simulink model "bObserver"  (R2020a)
settings: Solver=VariableStepAuto  StartTime=0.0  StopTime=1.5  FixedStep=0.0005  EnableMultiTasking=on
InitFcn:
  | kp=0.01;
  | ki=0.01;
  | 
  | k=2;
  | em=100000000;
  | GE=1/em;
  | GU=k*ki/GE;
  | GCE=k*kp/GU;
model workspace (MAT data in the model file):
  time = 0.8
values from neighbouring files (symbols this model uses):
  A1 = obj.boostConverter.A1    [BoostController.m]    (also in BoostConverter.m = [-obj.R/obj.L 0;0 -1/(obj.Ro*obj.C)]; BuckBoostConverter.m = [-obj.R/obj.L 0;0 -1/(obj.Ro*obj.C)]; obsmc.m = Asigma{1,1}; workspace_atual.mat = [-16.4  0; 0  -3.50877192982])
  A2 = obj.boostConverter.A2    [BoostController.m]    (also in BoostConverter.m = [-obj.R/obj.L -1/obj.L;1/obj.C -1/(obj.Ro*obj.C)]; BuckBoostConverter.m = [-obj.R/obj.L 1/obj.L;-1/obj.C -1/(obj.Ro*obj.C)]; obsmc.m = Asigma{1,2}; workspace_atual.mat = [-16.4  -200; 350.877192982  -3.50877192982])
  AlarmDeadTime = 0.50    (= 0.5)    [BoostFaultSimulation.m]    (also in workspace_atual.mat; workspace_certo.mat)
  B1 = obj.boostConverter.B1    [BoostController.m]    (also in BoostConverter.m = [1/obj.L;0]; BuckBoostConverter.m = [1/obj.L;0]; obsmc.m = Bsigma{1,1}; workspace_atual.mat = [200 0])
  B1f = [200 0]    [workspace_atual.mat]    (also in workspace_certo.mat)
  B2 = obj.boostConverter.B2    [BoostController.m]    (also in BoostConverter.m = obj.B1; obsmc.m = Bsigma{1,2}; workspace_atual.mat = [200 0]; workspace_certo.mat = [200 0])
  B2f = [200 0]    [workspace_atual.mat]    (also in workspace_certo.mat)
  boost_Amatrices = cat(3,obj.A1,obj.A2)    [BoostConverter.m]    (also in BuckBoostConverter.m; boostResults2Latex.m = boost.A_matrices(); workspace_atual.mat = [-16.4 0 0 -3.50877192982 -16.4 350.877192982 -200 -3.508771; workspace_certo.mat = [-16.4 0 0 -3.50877192982 -16.4 350.877192982 -200 -3.508771)
  boost_parameters = [obj.Ro,obj.R,obj.L,obj.C,obj.u]'    [BoostConverter.m]    (also in BuckBoostConverter.m; boostResults2Latex.m = boost.parameters(); workspace_atual.mat = [100 0.082 0.005 0.00285 190]; workspace_certo.mat = [100 0.082 0.005 0.00285 190])
  C = 1e-3    (= 0.001)    [boostResults2Latex.m]
  CiL = [0 1]    [workspace_atual.mat]    (also in workspace_certo.mat)
  Cmatrix = [1  0; 0  1]    [workspace_atual.mat]    (also in workspace_certo.mat)
  CVc = [1 0]    [workspace_atual.mat]    (also in workspace_certo.mat)
  D1 = [1  0; 0  1]    [workspace_atual.mat]    (also in workspace_certo.mat)
  F_11 = -16.4    [workspace_atual.mat]    (also in workspace_certo.mat)
  F_12 = -4812476.87956    [workspace_atual.mat]    (also in workspace_certo.mat)
  F_21 = -3.50877192982    [workspace_atual.mat]    (also in workspace_certo.mat)
  F_22 = -2.00703596657    [workspace_atual.mat]    (also in workspace_certo.mat)
  FaultClass = 0    [BoostFaultSimulation.m]    (also in workspace_atual.mat = 1; workspace_certo.mat = 1)
  H_1 = 13715.5123667    [workspace_atual.mat]    (also in workspace_certo.mat)
  iLFaultSwitch = 0    [BoostFaultSimulation.m]    (also in workspace_atual.mat; workspace_certo.mat)
  iLFaultTime = 1.70    (= 1.7)    [BoostFaultSimulation.m]    (also in workspace_atual.mat; workspace_certo.mat)
  iLGainFaultFactor = 15    [BoostFaultSimulation.m]    (also in workspace_atual.mat; workspace_certo.mat)
  iLNoiseFaultSwitch = 0    [BoostFaultSimulation.m]    (also in workspace_atual.mat; workspace_certo.mat)
  iLNoiseTime = 1.70    (= 1.7)    [BoostFaultSimulation.m]    (also in workspace_atual.mat; workspace_certo.mat)
  Jth = 2000    [workspace_atual.mat]    (also in workspace_certo.mat)
  L = 1e-3    (= 0.001)    [boostResults2Latex.m]    (also in obsmc.m = sdpvar(3,1,'full'))
  L_11 = -176809.798019    [workspace_atual.mat]    (also in workspace_certo.mat)
  L_12 = -66005538231.6    [workspace_atual.mat]    (also in workspace_certo.mat)
  L_21 = 0.0967961040176    [workspace_atual.mat]    (also in workspace_certo.mat)
  L_22 = 350.985265141    [workspace_atual.mat]    (also in workspace_certo.mat)
  LoadAddSignalSwitch = 1    [BoostFaultSimulation.m]    (also in workspace_atual.mat; workspace_certo.mat)
  LoadAddSwitch = 0    [BoostFaultSimulation.m]    (also in workspace_atual.mat; workspace_certo.mat)
  LoadAddTime = 0.90    (= 0.9)    [BoostFaultSimulation.m]    (also in workspace_atual.mat; workspace_certo.mat)
  LoadRemoveSignalSwitch = 1    [BoostFaultSimulation.m]    (also in workspace_atual.mat; workspace_certo.mat)
  LoadRemoveSwitch = 0    [BoostFaultSimulation.m]    (also in workspace_atual.mat; workspace_certo.mat)
  LoadRemoveTime = 0.90    (= 0.9)    [BoostFaultSimulation.m]    (also in workspace_atual.mat; workspace_certo.mat)
  LobsiL = [1737913.15707 66180.0912281]    [workspace_atual.mat]    (also in workspace_certo.mat)
  LobsVc = [61200 1]    [workspace_atual.mat]    (also in workspace_certo.mat)
  ObsEp = 70    [workspace_atual.mat]    (also in workspace_certo.mat)
  P = value(P)    [BoostController.m]    (also in boostResults2Latex.m = boost.calculateP(); obsmc.m = blkdiag(1/deltaAtilde(1,2),-1/deltaAtilde(2,1),1); workspace_atual.mat = [0.00235275094895  5.25738510027e-05; 5.25738510027e-05  0.0; workspace_certo.mat = [0.00235275094893  5.25738512446e-05; 5.25738512446e-05  0.0)
  Q_1 = [13715.5123667  1; 1  0]    [workspace_atual.mat]    (also in workspace_certo.mat)
  Q_2 = [1  0; 0.00750867981628  1]    [workspace_atual.mat]    (also in workspace_certo.mat)
  R = 0.1    [boostResults2Latex.m]    (also in workspace_atual.mat = 0.082; workspace_certo.mat = 0.082)
  ReconfigSwitch = 0    [BoostFaultSimulation.m]    (also in workspace_atual.mat; workspace_certo.mat)
  ReconfigTime = 1.707    [BoostFaultSimulation.m]    (also in workspace_atual.mat; workspace_certo.mat)
  rho = 5    [workspace_atual.mat]    (also in workspace_certo.mat)
  RMSfrequency = 47.61    [BoostFaultSimulation.m]    (also in workspace_atual.mat; workspace_certo.mat)
  Ro = 100    [BoostFaultSimulation.m]    (also in boostResults2Latex.m = 10; workspace_atual.mat; workspace_certo.mat)
  Smep = 80    [workspace_atual.mat]    (also in workspace_certo.mat)
  SourceAddSignalSwitch = 1    [BoostFaultSimulation.m]    (also in workspace_atual.mat; workspace_certo.mat)
  SourceAddSwitch = 0    [BoostFaultSimulation.m]    (also in workspace_atual.mat; workspace_certo.mat)
  SourceAddTime = 0.90    (= 0.9)    [BoostFaultSimulation.m]    (also in workspace_atual.mat; workspace_certo.mat)
  SourceAddVoltage = obj.SourceAddFactor*obj.u    [BoostFaultSimulation.m]    (also in workspace_atual.mat = 19; workspace_certo.mat = 19)
  SourceRemoveSignalSwitch = 1    [BoostFaultSimulation.m]    (also in workspace_atual.mat; workspace_certo.mat)
  SourceRemoveSwitch = 0    [BoostFaultSimulation.m]    (also in workspace_atual.mat; workspace_certo.mat)
  SourceRemoveTime = 0.90    (= 0.9)    [BoostFaultSimulation.m]    (also in workspace_atual.mat; workspace_certo.mat)
  SourceRemoveVoltage = obj.SourceRemoveFactor*obj.u    [BoostFaultSimulation.m]    (also in workspace_atual.mat = 19; workspace_certo.mat = 19)
  T_1 = [1 -13715.5123667]    [workspace_atual.mat]    (also in workspace_certo.mat)
  T_2 = [-0.00750867981628 1]    [workspace_atual.mat]    (also in workspace_certo.mat)
  ueq = 0.5    [workspace_atual.mat]    (also in workspace_certo.mat)
  uf = 190    [workspace_atual.mat]    (also in workspace_certo.mat)
  VcFaultSwitch = 0    [BoostFaultSimulation.m]    (also in workspace_atual.mat; workspace_certo.mat)
  VcFaultTime = 1.70    (= 1.7)    [BoostFaultSimulation.m]    (also in workspace_atual.mat; workspace_certo.mat)
  VcGainFaultFactor = 15    [BoostFaultSimulation.m]    (also in workspace_atual.mat; workspace_certo.mat)
  VcNoiseFaultSwitch = 0    [BoostFaultSimulation.m]    (also in workspace_atual.mat; workspace_certo.mat)
  VcNoiseTime = 1.70    (= 1.7)    [BoostFaultSimulation.m]    (also in workspace_atual.mat; workspace_certo.mat)
  ve = 380    [BoostFaultSimulation.m]    (also in boostResults2Latex.m = 100; workspace_atual.mat; workspace_certo.mat)
  x_e = [ie;ve]    [BoostConverter.m]    (also in BuckBoostConverter.m)
  xe = obj.boostConverter.equilibriumstate(ve)    [BoostController.m]    (also in workspace_atual.mat = [7.62509288104 380]; workspace_certo.mat = [7.62509288104 380])
undefined symbols (not defined in the file or in its folder): Atilde1, Atilde2, B1u, Ctilde1, Dtilde1, Dtilde2, F, F1, G, G1, MAXnet, MINnet
libraries: neural x36, powerlib x34, dspstat3 x11, PhdLibrary x10, simulink x7, dspmtrx3 x6, powerlib_meascontrol x4, dspmathops x4
(part 3 of 6)

== system bObserver/ROSLSO/Bank of ROSLSO/z1 ==
  y_f1 : Inport
  sigma : Inport  Port=2
  Constant : Constant  Value=F_11  VectorParams1D=off
  Constant10 : Constant  Value=T_1  VectorParams1D=off
  Constant2 : Constant  Value=F_12  VectorParams1D=off
  Constant4 : Constant  Value=L_11  VectorParams1D=off
  Constant5 : Constant  Value=L_12  VectorParams1D=off
  Integral : Subsystem
  Matrix Multiply{,1..4} (5 alike) : Product  Multiplication=Matrix(*)
  MatrizesA8 : Constant  Value=B1u  VectorParams1D=off
  Sum : Sum  Inputs=|+++
  Sum1 : Sum  Inputs=|+++
  Switch1 : Switch  Criteria=u2 ~= 0
  z : Outport
  wires:
  sigma/1 -> Switch1/2
  Switch1/1 -> Integral/1(z_dot)  "z"
  Sum/1 -> [sys1]
  Sum1/1 -> [sys2]
  Integral/1(z) -> [z], z/1
  y_f1/1 -> Matrix Multiply2/2, Matrix Multiply/2
  MatrizesA8/1 -> Matrix Multiply1/2
  Constant10/1 -> Matrix Multiply1/1
  Matrix Multiply1/1 -> [TBu]
  Matrix Multiply/1 -> [Ly1]
  Matrix Multiply2/1 -> [Ly2]
  Matrix Multiply3/1 -> [Fz1]
  Constant/1 -> Matrix Multiply3/1
  Matrix Multiply4/1 -> [Fz2]
  Constant2/1 -> Matrix Multiply4/1
  [z] -> Matrix Multiply4/2
  [Fz1] -> Sum/1
  [Fz2] -> Sum1/1
  [z] -> Matrix Multiply3/2
  [sys1] -> Switch1/1
  [sys2] -> Switch1/3
  [TBu] -> Sum/2
  [TBu] -> Sum1/2
  [Ly2] -> Sum1/3
  [Ly1] -> Sum/3
  Constant4/1 -> Matrix Multiply/1
  Constant5/1 -> Matrix Multiply2/1

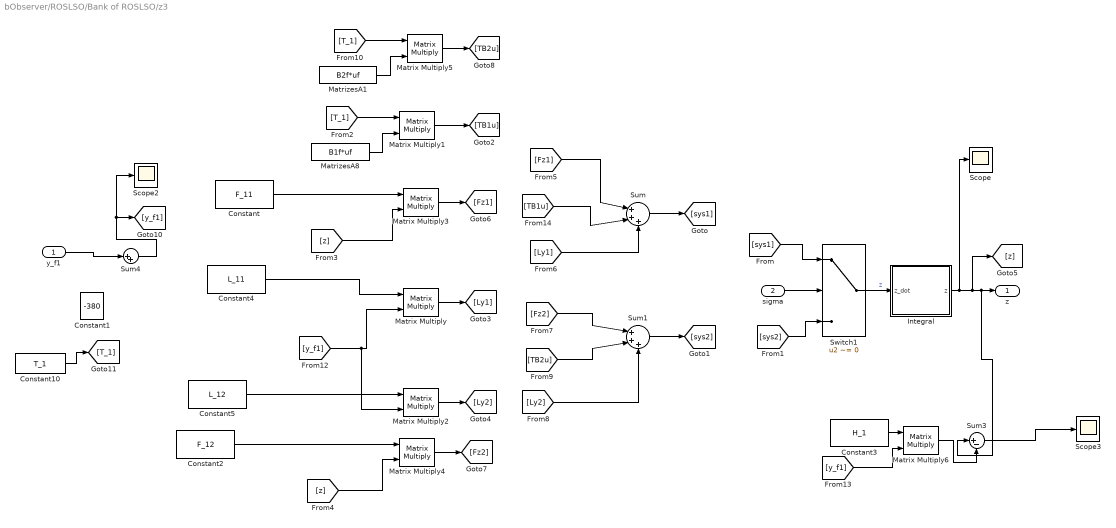
== system bObserver/ROSLSO/Bank of ROSLSO/z3 ==
  y_f1 : Inport
  sigma : Inport  Port=2
  Constant : Constant  Value=F_11  VectorParams1D=off
  Constant1 : Constant  Value=-380
  Constant10 : Constant  Value=T_1  VectorParams1D=off
  Constant2 : Constant  Value=F_12  VectorParams1D=off
  Constant3 : Constant  Value=H_1  VectorParams1D=off
  Constant4 : Constant  Value=L_11  VectorParams1D=off
  Constant5 : Constant  Value=L_12  VectorParams1D=off
  Integral : Subsystem
  Matrix Multiply{,1..6} (7 alike) : Product  Multiplication=Matrix(*)
  MatrizesA1 : Constant  Value=B2f*uf  VectorParams1D=off
  MatrizesA8 : Constant  Value=B1f*uf  VectorParams1D=off
  Scope : Scope
  Scope2 : Scope
  Scope3 : Scope
  Sum : Sum  Inputs=|+++
  Sum1 : Sum  Inputs=|+++
  Sum3 : Sum  Inputs=|+-
  Sum4 : Sum  Inputs=|++
  Switch1 : Switch  Criteria=u2 ~= 0
  z : Outport
  wires:
  sigma/1 -> Switch1/2
  Switch1/1 -> Integral/1(z_dot)  "z"
  Sum/1 -> [sys1]
  Sum1/1 -> [sys2]
  Integral/1(z) -> Scope/1, [z], Sum3/1, z/1
  MatrizesA8/1 -> Matrix Multiply1/2
  [T_1] -> Matrix Multiply1/1
  Matrix Multiply1/1 -> [TB1u]
  Matrix Multiply/1 -> [Ly1]
  Matrix Multiply2/1 -> [Ly2]
  Matrix Multiply3/1 -> [Fz1]
  Matrix Multiply4/1 -> [Fz2]
  [z] -> Matrix Multiply4/2
  [Fz1] -> Sum/1
  [Fz2] -> Sum1/1
  [z] -> Matrix Multiply3/2
  [sys1] -> Switch1/1
  [sys2] -> Switch1/3
  [TB2u] -> Sum1/2
  [Ly2] -> Sum1/3
  [Ly1] -> Sum/3
  Constant4/1 -> Matrix Multiply/1
  Constant3/1 -> Matrix Multiply6/1
  [y_f1] -> Matrix Multiply2/2, Matrix Multiply/2
  [y_f1] -> Matrix Multiply6/2
  Matrix Multiply6/1 -> Sum3/2
  Sum3/1 -> Scope3/1
  Constant/1 -> Matrix Multiply3/1
  Constant2/1 -> Matrix Multiply4/1
  Constant5/1 -> Matrix Multiply2/1
  y_f1/1 -> Sum4/1
  Sum4/1 -> Scope2/1, [y_f1]
  [TB1u] -> Sum/2
  Constant10/1 -> [T_1]
  [T_1] -> Matrix Multiply5/1
  Matrix Multiply5/1 -> [TB2u]
  MatrizesA1/1 -> Matrix Multiply5/2

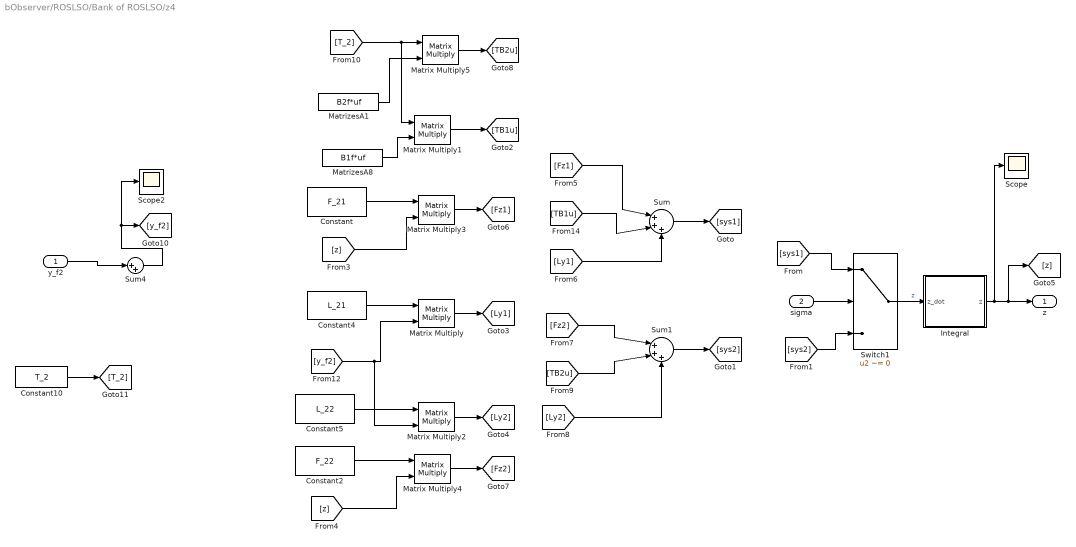
== system bObserver/ROSLSO/Bank of ROSLSO/z4 ==
  y_f2 : Inport
  sigma : Inport  Port=2
  Constant : Constant  Value=F_21  VectorParams1D=off
  Constant10 : Constant  Value=T_2  VectorParams1D=off
  Constant2 : Constant  Value=F_22  VectorParams1D=off
  Constant4 : Constant  Value=L_21  VectorParams1D=off
  Constant5 : Constant  Value=L_22  VectorParams1D=off
  Integral : Subsystem
  Matrix Multiply{,1..5} (6 alike) : Product  Multiplication=Matrix(*)
  MatrizesA1 : Constant  Value=B2f*uf  VectorParams1D=off
  MatrizesA8 : Constant  Value=B1f*uf  VectorParams1D=off
  Scope : Scope
  Scope2 : Scope
  Sum : Sum  Inputs=|+++
  Sum1 : Sum  Inputs=|+++
  Sum4 : Sum  Inputs=|++
  Switch1 : Switch  Criteria=u2 ~= 0
  z : Outport
  wires:
  sigma/1 -> Switch1/2
  Switch1/1 -> Integral/1(z_dot)  "z"
  Sum/1 -> [sys1]
  Sum1/1 -> [sys2]
  Integral/1(z) -> Scope/1, [z], z/1
  MatrizesA8/1 -> Matrix Multiply1/2
  [T_2] -> Matrix Multiply1/1, Matrix Multiply5/1
  Matrix Multiply1/1 -> [TB1u]
  Matrix Multiply/1 -> [Ly1]
  Matrix Multiply2/1 -> [Ly2]
  Matrix Multiply3/1 -> [Fz1]
  Matrix Multiply4/1 -> [Fz2]
  [z] -> Matrix Multiply4/2
  [Fz1] -> Sum/1
  [Fz2] -> Sum1/1
  [z] -> Matrix Multiply3/2
  [sys1] -> Switch1/1
  [sys2] -> Switch1/3
  Constant4/1 -> Matrix Multiply/1
  [y_f2] -> Matrix Multiply2/2, Matrix Multiply/2
  Constant/1 -> Matrix Multiply3/1
  Constant2/1 -> Matrix Multiply4/1
  Constant5/1 -> Matrix Multiply2/1
  y_f2/1 -> Sum4/1
  Sum4/1 -> Scope2/1, [y_f2]
  Constant10/1 -> [T_2]
  Matrix Multiply5/1 -> [TB2u]
  MatrizesA1/1 -> Matrix Multiply5/2
  [TB1u] -> Sum/2
  [TB2u] -> Sum1/2
  [Ly1] -> Sum/3
  [Ly2] -> Sum1/3

== system bObserver/ROSLSO/Bank of ROSMO/Subsystem ==
  y : Inport
  C : Inport  Port=2
  y_hat : Inport  Port=3
  "    1" : Constant  Value=ObsEp
  Product : Product  Multiplication=Matrix(*)
  SlidingSurface : Subsystem
  Subtract : Sum  Inputs=+-
  error : Outport
  wires:
  Subtract/1 -> SlidingSurface/1(S)  "y-y_hat"
  Product/1 -> Subtract/1
  "    1"/1 -> SlidingSurface/2(ep)
  SlidingSurface/1(d) -> error/1
  y_hat/1 -> Subtract/2
  C/1 -> Product/1
  y/1 -> Product/2

== system bObserver/ROSLSO/Bank of ROSMO/Subsystem1 ==
  y : Inport
  C : Inport  Port=2
  y_hat : Inport  Port=3
  "    1" : Constant  Value=ObsEp
  Product : Product  Multiplication=Matrix(*)
  SlidingSurface : Subsystem
  Subtract : Sum  Inputs=+-
  error : Outport
  wires:
  Subtract/1 -> SlidingSurface/1(S)  "y-y_hat"
  Product/1 -> Subtract/1
  "    1"/1 -> SlidingSurface/2(ep)
  SlidingSurface/1(d) -> error/1
  y_hat/1 -> Subtract/2
  C/1 -> Product/1
  y/1 -> Product/2

== system bObserver/ROSLSO/Bank of ROSMO/Vc OBserver ==
  ObserverError : Inport
  C : Inport  Port=2
  sigma : Inport  Port=3
  Constant : Constant  Value=LobsVc
  Product2 : Product  Multiplication=Matrix(*)
  calc_x_hat : Subsystem
  x_hat : Outport
  y_hat : Outport  Port=2
  wires:
  sigma/1 -> calc_x_hat/1(sigma)
  calc_x_hat/1(x_hat) -> Product2/2, x_hat/1
  Product2/1 -> y_hat/1
  C/1 -> Product2/1
  ObserverError/1 -> calc_x_hat/2(rsign)
  Constant/1 -> calc_x_hat/3(Lobs)

== system bObserver/ROSLSO/Bank of ROSMO/iL Observer ==
  C : Inport
  ObserverError : Inport  Port=2
  sigma : Inport  Port=3
  Constant8 : Constant  Value=LobsiL
  Product2 : Product  Multiplication=Matrix(*)
  calc_x_hat : Subsystem
  x_hat : Outport
  y_hat : Outport  Port=2
  wires:
  sigma/1 -> calc_x_hat/1(sigma)
  calc_x_hat/1(x_hat) -> Product2/2, x_hat/1
  Product2/1 -> y_hat/1
  C/1 -> Product2/1
  ObserverError/1 -> calc_x_hat/2(rsign)
  Constant8/1 -> calc_x_hat/3(Lobs)

== system bObserver/ROSLSO/Boost Converter/Integral ==
  x_dot : Inport
  Ground : Ground
  Ground1 : Ground
  IC : InitialCondition  Value=[0;0]
  Integrator1 : Integrator  InitialConditionSource=external  InitialCondition=[-x_e; 0; 0]
  Mux : Mux  Inputs=2
  x : Outport
  wires:
  x_dot/1 -> Integrator1/1
  Integrator1/1 -> x/1
  IC/1 -> Integrator1/2
  Ground1/1 -> Mux/2
  Ground/1 -> Mux/1
  Mux/1 -> IC/1

== system bObserver/ROSLSO/Chaveado_fixo1/Controlador Chavead ==
  Ve : Inport
  x : Inport  Port=2
  MatirxControle : Subsystem
  Matrix P : Constant  Value=P
  Matrizes A : Constant  Value=boost_Amatrices
  Parametros do Boost : Constant  Value=boost_parameters
  sigma : Outport
  x_e : Outport  Port=2
  i_e : Outport  Port=3
  wires:
  Parametros do Boost/1 -> MatirxControle/1("boost_parameters ")
  Matrizes A/1 -> MatirxControle/2(boost_Amatrices)
  Matrix P/1 -> MatirxControle/3(P)
  x/1 -> MatirxControle/5(x)
  Ve/1 -> MatirxControle/4(ve)
  MatirxControle/1(sigma) -> sigma/1
  MatirxControle/2(x_e) -> x_e/1
  MatirxControle/3(i_e) -> i_e/1

== system bObserver/ROSLSO/Controlador1/SlidingSurface ==
  S : Inport
  ep : Inport  Port=2
  Abs : Abs
  GreaterThan : RelationalOperator  Operator=>  OutDataTypeStr=boolean  RndMeth=Simplest
  If : If  IfExpression=u1 ~= 0
  If Action Subsystem : Subsystem  TreatAsAtomicUnit=on
  If Action Subsystem2 : Subsystem  TreatAsAtomicUnit=on
  Merge1 : Merge
  d : Outport
  wires:
  If Action Subsystem2/1(d) -> Merge1/2
  [S] -> If Action Subsystem/1(S), If Action Subsystem2/1(S)
  If/2 -> If Action Subsystem2/Action
  If/1 -> If Action Subsystem/Action
  [ep] -> If Action Subsystem2/2(ep)
  S/1 -> [S], Abs/1
  If Action Subsystem/1(d) -> Merge1/1
  Abs/1 -> GreaterThan/1
  GreaterThan/1 -> If/1
  Merge1/1 -> d/1
  ep/1 -> [ep], GreaterThan/2

== system bObserver/ROSLSO/Fault Diagnostics/AntiFalseAlarm ==
  PRNN : Inport
  Alarm : Inport  Port=2
  Constant7 : Constant
  FaultDetecition1 : Switch  Criteria=u2 > Threshold
  Product1 : Product
  Step1 : Step  Time=AlarmDeadTime  SampleTime=0
  FaultClass : Outport
  AlarmOut : Outport  Port=2
  wires:
  PRNN/1 -> FaultDetecition1/1
  Constant7/1 -> FaultDetecition1/3
  Step1/1 -> Product1/1
  Alarm/1 -> Product1/2
  FaultDetecition1/1 -> FaultClass/1
  Product1/1 -> AlarmOut/1, FaultDetecition1/2

== system bObserver/ROSLSO/Fault Diagnostics/Augmented Error Generator ==
  e : Inport
  Mux : Mux  Inputs=2
  z1 : Subsystem
  e_tilde : Outport
  wires:
  z1/1(z) -> Mux/2
  Mux/1 -> e_tilde/1
  e/1 -> Mux/1, z1/1(z_dot)

== system bObserver/ROSLSO/Fault Diagnostics/ErrorGenerator ==
  y_e_tilde : Inport
  y_e_tilde_hat : Inport  Port=2
  AND : Logic  IconShape=distinctive  AllPortsSameDT=off  OutDataTypeStr=boolean
  Compare To Zero : simulink/Logic and Bit Operations/Compare To Zero  relop=~=  OutDataTypeStr=boolean
  Constant1 : Constant  Value=[0;0]
  Demux : Demux  Outputs=2
  If : If  IfExpression=u1 ~= 0
  If Action Subsystem : Subsystem  TreatAsAtomicUnit=on
  If Action Subsystem1 : Subsystem  TreatAsAtomicUnit=on
  Merge : Merge  InitialOutput=[0;0]
  Sum : Sum  Inputs=|+-
  e_y : Outport
  v : Outport  Port=2
  wires:
  y_e_tilde/1 -> Sum/1
  y_e_tilde_hat/1 -> Sum/2
  Sum/1 -> Compare To Zero/1, e_y/1, [e_y]
  If/1 -> If Action Subsystem/Action
  If/2 -> If Action Subsystem1/Action
  [e_y] -> If Action Subsystem/1(e_y)
  Constant1/1 -> If Action Subsystem1/1(e_y)
  If Action Subsystem/1(v) -> Merge/1
  If Action Subsystem1/1(v) -> Merge/2
  Demux/1 -> AND/1
  Demux/2 -> AND/2
  AND/1 -> If/1
  Merge/1 -> v/1
  Compare To Zero/1 -> Demux/1

== system bObserver/ROSLSO/Fault Diagnostics/Fault Identification Neural Netowrk ==
  netInputs : Inport
  Constant : Constant  Commented=on  Value=MAXnet
  Constant1 : Constant  Commented=on  Value=[0;0;0]
  Constant4 : Constant  Commented=on  Value=MINnet
  Demux : Demux  Commented=on  Outputs=3
  Demux1 : Demux  Commented=on  Outputs=3
  Demux2 : Demux  Commented=on  Outputs=3
  Maximum : dspstat3/Maximum  operation=maximum  fcn=Value and Index  indexBase=One  operateOver=Each column  Dimension=1  InputProcessing=Columns as channels (frame based)  reset=None  roiEnable=off  roiType=Rectangles  roiPortion=Entire ROI  roiOutput=Individual statistics for each ROI  roiFlag=off  roundingMode=Floor  overflowMode=off  accumDataTypeStr=Inherit: Same as product output  accumLastDataTypeStr=Inherit: Same as product output
  Median Filter : dspstat3/Median Filter  Commented=on  WindowLength=1  SimulateUsing=Code generation
      settings: SourceProductBaseCode=DS
  Mux : Mux  Commented=on  Inputs=3
  Pattern Recognition Neural Network1 : Subsystem
      mask help: Pattern Recognition Neural Network
      mask Display: e = 0.06;c1 = [120 150 230]/255;c2 = ([120 150 230]+0)/383;c3 = ([120 150 230]+128)/383;patch([0 1 1 0],[0 0 1 1],c1);patch([0 1 1 1-e 1-e 0+e],[0 0 1 1-e 0+e 0+e],c2);patch([0 0 1 1-e 0+e 0+e],[0 1 1 1-e 1-e 0+e],c3);plot([0 1 1 0 0],[0 0 1 1 0]);fprintf('NNET');port_label('input',1,' Input');port_label('output',1,'Output ');
  Scope : Scope
  Scope1 : Scope
  Subsystem : Subsystem  Commented=on
  Subsystem1 : Subsystem  Commented=on
  Subsystem2 : Subsystem  Commented=on
  Terminator : Terminator
  netOutputs : Outport
  wires:
  Maximum/1 -> Terminator/1
  Maximum/2 -> Scope1/1, netOutputs/1, Scope/1
  Constant/1 -> Demux/1
  Demux2/1 -> Subsystem/1(input)
  Demux1/1 -> Subsystem/2(min)
  Demux/1 -> Subsystem/3(max)
  Demux1/2 -> Subsystem1/2(min)
  Demux/2 -> Subsystem1/3(max)
  Demux2/2 -> Subsystem1/1(input)
  Demux/3 -> Subsystem2/3(max)
  Demux1/3 -> Subsystem2/2(min)
  Demux2/3 -> Subsystem2/1(input)
  Subsystem/1(Out1) -> Mux/1
  Subsystem1/1(Out1) -> Mux/2
  Subsystem2/1(Out1) -> Mux/3
  Constant4/1 -> Demux1/1
  netInputs/1 -> Pattern Recognition Neural Network1/1(Input)
  Pattern Recognition Neural Network1/1(Output) -> Maximum/1

== system bObserver/ROSLSO/Fault Diagnostics/Residual Generator2 ==
  e_y : Inport
  Matrix Square1 : dspmtrx3/Matrix Square  OutMin=[]  OutMax=[]
      settings: SourceProductBaseCode=DS
  Moving RMS : dspstat3/Moving RMS  Method=Sliding window  ForgettingFactorPort=off  SpecifyWindowLength=on  WindowLength=RMSfrequency/10  ForgettingFactor=0.9  SimulateUsing=Code generation
      settings: SourceProductBaseCode=DS
  Sqrt2 : Sqrt  SaturateOnIntegerOverflow=on
  RMS : Outport
  wires:
  Matrix Square1/1 -> Sqrt2/1
  e_y/1 -> Matrix Square1/1
  Sqrt2/1 -> Moving RMS/1
  Moving RMS/1 -> RMS/1

== system bObserver/ROSLSO/Fault Diagnostics/Sliding Mode Observer 5 ==
  ey : Inport
  v : Inport  Port=2
  sigma : Inport  Port=3
  C : Constant  Value=Ctilde1
  ObserverDynamics : Subsystem
  Product : Product  Multiplication=Matrix(*)
  ey_out : Outport
  y_e_tilde_hat : Outport  Port=2
  wires:
  Product/1 -> y_e_tilde_hat/1
  C/1 -> Product/1
  ObserverDynamics/1(e_tilde_hat) -> Product/2
  sigma/1 -> ObserverDynamics/3(sigma)
  ey/1 -> ey_out/1, ObserverDynamics/1(ey)
  v/1 -> ObserverDynamics/2(v)

== system bObserver/ROSLSO/Fault Diagnostics/Subsystem9 ==
  x : Inport
  Demux : Demux  Outputs=2
  Residual Generator2 : Subsystem
  Terminator : Terminator
  VcRMS : Outport
  wires:
  x/1 -> Demux/1
  Demux/2 -> Residual Generator2/1(e_y)
  Residual Generator2/1(RMS) -> VcRMS/1
  Demux/1 -> Terminator/1

== system bObserver/ROSMO_L1/Augmented Error Generator/z1 ==
  z_dot : Inport
  Constant1 : Constant  Value=[0;0]  VectorParams1D=off
  Gain2 : Gain  Gain=Cmatrix  Multiplication=Matrix(K*u) (u vector)
  Integrator6 : Integrator  InitialConditionSource=external
  z : Outport
  wires:
  Gain2/1 -> Integrator6/1
  Integrator6/1 -> z/1
  z_dot/1 -> Gain2/1
  Constant1/1 -> Integrator6/2

== system bObserver/ROSMO_L1/Boost Converter/Integral ==
  x_dot : Inport
  Ground : Ground
  Ground1 : Ground
  IC : InitialCondition  Value=[0;0]
  Integrator1 : Integrator  InitialConditionSource=external  InitialCondition=[-x_e; 0; 0]
  Mux : Mux  Inputs=2
  x : Outport
  wires:
  x_dot/1 -> Integrator1/1
  Integrator1/1 -> x/1
  IC/1 -> Integrator1/2
  Ground1/1 -> Mux/2
  Ground/1 -> Mux/1
  Mux/1 -> IC/1

== system bObserver/ROSMO_L1/Controlador2/SlidingSurface ==
  S : Inport
  ep : Inport  Port=2
  Abs : Abs
  GreaterThan : RelationalOperator  Operator=>  OutDataTypeStr=boolean  RndMeth=Simplest
  If : If  IfExpression=u1 ~= 0
  If Action Subsystem : Subsystem  TreatAsAtomicUnit=on
  If Action Subsystem2 : Subsystem  TreatAsAtomicUnit=on
  Merge1 : Merge
  d : Outport
  wires:
  If Action Subsystem2/1(d) -> Merge1/2
  [S] -> If Action Subsystem/1(S), If Action Subsystem2/1(S)
  If/2 -> If Action Subsystem2/Action
  If/1 -> If Action Subsystem/Action
  [ep] -> If Action Subsystem2/2(ep)
  S/1 -> [S], Abs/1
  If Action Subsystem/1(d) -> Merge1/1
  Abs/1 -> GreaterThan/1
  GreaterThan/1 -> If/1
  Merge1/1 -> d/1
  ep/1 -> [ep], GreaterThan/2

== system bObserver/ROSMO_L1/SMO/ErrorGenerator ==
  y_e_tilde : Inport
  y_e_tilde_hat : Inport  Port=2
  AND : Logic  IconShape=distinctive  AllPortsSameDT=off  OutDataTypeStr=boolean
  Compare To Zero : simulink/Logic and Bit Operations/Compare To Zero  relop=~=  OutDataTypeStr=boolean
  Constant1 : Constant  Value=[0;0]
  Demux : Demux  Outputs=2
  If : If  IfExpression=u1 ~= 0
  If Action Subsystem : Subsystem  TreatAsAtomicUnit=on
  If Action Subsystem1 : Subsystem  TreatAsAtomicUnit=on
  Merge : Merge  InitialOutput=[0;0]
  Sum : Sum  Inputs=|+-
  e_y : Outport
  v : Outport  Port=2
  wires:
  y_e_tilde/1 -> Sum/1
  y_e_tilde_hat/1 -> Sum/2
  Sum/1 -> Compare To Zero/1, e_y/1, [e_y]
  If/1 -> If Action Subsystem/Action
  If/2 -> If Action Subsystem1/Action
  [e_y] -> If Action Subsystem/1(e_y)
  Constant1/1 -> If Action Subsystem1/1(e_y)
  If Action Subsystem/1(v) -> Merge/1
  If Action Subsystem1/1(v) -> Merge/2
  Demux/1 -> AND/1
  Demux/2 -> AND/2
  AND/1 -> If/1
  Merge/1 -> v/1
  Compare To Zero/1 -> Demux/1

== system bObserver/ROSMO_L1/SMO/Sliding Mode Observer 5 ==
  ey : Inport
  v : Inport  Port=2
  sigma : Inport  Port=3
  C : Constant  Value=Ctilde1
  ObserverDynamics : Subsystem
  Product : Product  Multiplication=Matrix(*)
  ey_out : Outport
  y_e_tilde_hat : Outport  Port=2
  wires:
  Product/1 -> y_e_tilde_hat/1
  C/1 -> Product/1
  ObserverDynamics/1(e_tilde_hat) -> Product/2
  sigma/1 -> ObserverDynamics/3(sigma)
  ey/1 -> ey_out/1, ObserverDynamics/1(ey)
  v/1 -> ObserverDynamics/2(v)

== system bObserver/ROSMO_ROSLSO/Augmented Error Generator/z1 ==
  z_dot : Inport
  Constant1 : Constant  Value=[0;0]  VectorParams1D=off
  Gain2 : Gain  Gain=Cmatrix  Multiplication=Matrix(K*u) (u vector)
  Integrator6 : Integrator  InitialConditionSource=external
  z : Outport
  wires:
  Gain2/1 -> Integrator6/1
  Integrator6/1 -> z/1
  z_dot/1 -> Gain2/1
  Constant1/1 -> Integrator6/2

== system bObserver/ROSMO_ROSLSO/Bank of ROSLSO/ROSLSO 2 Subsystems ==
  u : Inport
  y : Inport  Port=2
  sigma : Inport  Port=3
  Constant8 : Constant  Value=Q  VectorParams1D=off
  Integrator1 : Integrator  InitialCondition=z0
  Matrix Multiply6 : Product  Multiplication=Matrix(*)
  Mux : Mux  Inputs=2
  Reduced Order Derivate Z : Subsystem  mask(Reduced Order Observer Derivate Z){F=F1, L=L1, T=T, B=B1}
      mask prompts: F "Observer gain matrix:"; L "Output gain matrix:"; T "Input gain matrix:"; B "Input matrix:"
      mask help: Reduced Order Observer Derivate Z generates just zdot, without feedbak
  Reduced Order Derivate Z1 : Subsystem  mask(Reduced Order Observer Derivate Z){F=F2, L=L2, T=T, B=B2}
      mask prompts: F "Observer gain matrix:"; L "Output gain matrix:"; T "Input gain matrix:"; B "Input matrix:"
      mask help: Reduced Order Observer Derivate Z generates just zdot, without feedbak
  Switch1 : Switch  Criteria=u2 ~= 0
  z : Outport
  xhat : Outport  Port=2
  wires:
  sigma/1 -> Switch1/2
  Switch1/1 -> Integrator1/1  "zdot"
  y/1 -> [y]
  Constant8/1 -> Matrix Multiply6/1
  Matrix Multiply6/1 -> xhat/1
  Mux/1 -> Matrix Multiply6/2
  [y] -> Mux/1
  Reduced Order Derivate Z/1(zdot) -> Switch1/1
  u/1 -> Reduced Order Derivate Z1/1(u), Reduced Order Derivate Z/1(u)
  [y] -> Reduced Order Derivate Z1/2(y), Reduced Order Derivate Z/2(y)
  [z] -> Reduced Order Derivate Z/3(z), Reduced Order Derivate Z1/3(z)
  Reduced Order Derivate Z1/1(zdot) -> Switch1/3
  Integrator1/1 -> z/1, Mux/2, [z]

== system bObserver/ROSMO_ROSLSO/Bank of ROSLSO/ROSLSO 2 Subsystems1 ==
  u : Inport
  y : Inport  Port=2
  sigma : Inport  Port=3
  Constant8 : Constant  Value=Q  VectorParams1D=off
  Integrator1 : Integrator  InitialCondition=z0
  Matrix Multiply6 : Product  Multiplication=Matrix(*)
  Mux : Mux  Inputs=2
  Reduced Order Derivate Z : Subsystem  mask(Reduced Order Observer Derivate Z){F=F1, L=L1, T=T, B=B1}
      mask prompts: F "Observer gain matrix:"; L "Output gain matrix:"; T "Input gain matrix:"; B "Input matrix:"
      mask help: Reduced Order Observer Derivate Z generates just zdot, without feedbak
  Reduced Order Derivate Z1 : Subsystem  mask(Reduced Order Observer Derivate Z){F=F2, L=L2, T=T, B=B2}
      mask prompts: F "Observer gain matrix:"; L "Output gain matrix:"; T "Input gain matrix:"; B "Input matrix:"
      mask help: Reduced Order Observer Derivate Z generates just zdot, without feedbak
  Switch1 : Switch  Criteria=u2 ~= 0
  z : Outport
  xhat : Outport  Port=2
  wires:
  sigma/1 -> Switch1/2
  Switch1/1 -> Integrator1/1  "zdot"
  y/1 -> [y]
  Constant8/1 -> Matrix Multiply6/1
  Matrix Multiply6/1 -> xhat/1
  Mux/1 -> Matrix Multiply6/2
  [y] -> Mux/1
  Reduced Order Derivate Z/1(zdot) -> Switch1/1
  u/1 -> Reduced Order Derivate Z1/1(u), Reduced Order Derivate Z/1(u)
  [y] -> Reduced Order Derivate Z1/2(y), Reduced Order Derivate Z/2(y)
  [z] -> Reduced Order Derivate Z/3(z), Reduced Order Derivate Z1/3(z)
  Reduced Order Derivate Z1/1(zdot) -> Switch1/3
  Integrator1/1 -> z/1, Mux/2, [z]

== system bObserver/ROSMO_ROSLSO/Boost Converter/Integral ==
  x_dot : Inport
  Ground : Ground
  Ground1 : Ground
  IC : InitialCondition  Value=[0;0]
  Integrator1 : Integrator  InitialConditionSource=external  InitialCondition=[-x_e; 0; 0]
  Mux : Mux  Inputs=2
  x : Outport
  wires:
  x_dot/1 -> Integrator1/1
  Integrator1/1 -> x/1
  IC/1 -> Integrator1/2
  Ground1/1 -> Mux/2
  Ground/1 -> Mux/1
  Mux/1 -> IC/1

== system bObserver/ROSMO_ROSLSO/Boost Converter Circuit/Boost Converter Circuit ==
  sigma : Inport
  Ground : powerlib/Elements/Ground  LConnTagsString=a
  IGBT/Diode1 : powerlib/Power Electronics/IGBT//Diode  Ron=1e-3  Rs=1e5  Cs=inf  Measurements=on
  IL : powerlib/Measurements/Current Measurement  PhasorSimulation=off  OutputType=Complex  PSBequivalent=0
  Iro : powerlib/Measurements/Current Measurement  PhasorSimulation=off  OutputType=Complex  PSBequivalent=0
  R : powerlib/Elements/Series RLC Branch  LConnTagsString=__new0  RConnTagsString=__new0  BranchType=R  Resistance=R  Inductance=1e-3  SetiL0=off  InitialCurrent=0  Capacitance=1e-6  Setx0=off  InitialVoltage=0  Measurements=None
  S2 : powerlib/Power Electronics/Diode  Ron=0.000001  Lon=0  Vf=0  IC=0  UseSnubber=off  Rs=0  Cs=0  Measurements=on
  Terminator : Terminator
  Terminator4 : Terminator
  Voltage Measurement : powerlib/Measurements/Voltage Measurement  PhasorSimulation=off  OutputType=Complex  PSBequivalent=0
  c : powerlib/Elements/Series RLC Branch  LConnTagsString=__new0  RConnTagsString=__new0  BranchType=C  Resistance=1  Inductance=1e-3  SetiL0=off  InitialCurrent=0  Capacitance=C  Setx0=on  InitialVoltage=0  Measurements=None
  l : powerlib/Elements/Series RLC Branch  LConnTagsString=__new0  RConnTagsString=__new0  BranchType=L  Resistance=1  Inductance=L  SetiL0=on  InitialCurrent=0  Capacitance=1e-6  Setx0=off  InitialVoltage=0  Measurements=None
  V+ : PMIOPort  Side=Left
  V- : PMIOPort  Port=2  Side=Left
  Ro+ : PMIOPort  Port=3  Side=Left
  Ro- : PMIOPort  Port=4  Side=Left
  iL : Outport
  Vc : Outport  Port=2
  iro : Outport  Port=3
  wires:
  IL/1 -> iL/1
  sigma/1 -> IGBT/Diode1/1
  Voltage Measurement/1 -> Vc/1
  Iro/1 -> iro/1
  IGBT/Diode1/1 -> Terminator/1
  S2/1 -> Terminator4/1
  connections:
  IL/LConn1 -- l/RConn1
  c/RConn1 -- Ro-/RConn1 -- IGBT/Diode1/RConn1 -- V-/RConn1 -- Ground/LConn1 -- Voltage Measurement/LConn2
  S2/LConn1 -- IGBT/Diode1/LConn1 -- IL/RConn1
  l/LConn1 -- R/RConn1
  S2/RConn1 -- Iro/LConn1 -- c/LConn1 -- Voltage Measurement/LConn1
  V+/RConn1 -- R/LConn1
  Ro+/RConn1 -- Iro/RConn1

== system bObserver/ROSMO_ROSLSO/Boost Converter Circuit/DC Source ==
  Constant11 : Constant  Value=SourceRemoveSwitch
  Constant4 : Constant  Value=SourceAddSwitch
  Constant8 : Constant  Value=SourceRemoveSwitch
  Logical Operator : Logic  Operator=NOT  AllPortsSameDT=off  OutDataTypeStr=boolean
  Logical Operator3 : Logic  Operator=NOT  AllPortsSameDT=off  OutDataTypeStr=boolean
  Sen Disturbiio : Constant  Value=0
  Sen Disturbiio1 : Constant  Value=0
  Step Perturbation VAdd : PhdLibrary/Step Perturbation  SignalSwitch=SourceAddSignalSwitch  InitialMagnitude=0  InitialTime=SourceAddTime  Magnitude=1  Duration=0.1
      settings: SourceProductName=Phd Diego
  Step Perturbation VRemove : PhdLibrary/Step Perturbation  SignalSwitch=SourceRemoveSignalSwitch  InitialMagnitude=0  InitialTime=SourceRemoveTime  Magnitude=1  Duration=0.1
      settings: SourceProductName=Phd Diego
  Switch10 : Switch  Criteria=u2 ~= 0
  Switch8 : Switch  Criteria=u2 ~= 0
  Switch9 : Switch  Criteria=u2 ~= 0
  Variable DC Source : Subsystem  mask(Variable DC source){u=u, uAdd=SourceAddVoltage, uRemove=SourceRemoveVoltage}
      mask prompts: u "Input voltage:"; uAdd "Addtional voltage:"; uRemove "Voltage Reduction"
      mask help: Add or remove the source value acording to input signal
  V+ : PMIOPort  Side=Right
  V- : PMIOPort  Port=2  Side=Right
  wires:
  Sen Disturbiio1/1 -> Switch8/3
  Switch10/1 -> Logical Operator/1
  Sen Disturbiio/1 -> Switch10/3
  Switch8/1 -> Logical Operator3/1
  Logical Operator3/1 -> [VinputRemove]
  Logical Operator/1 -> [VinputAdd]
  Constant4/1 -> Switch10/2
  Constant8/1 -> Switch8/2
  [VinputRemove] -> Switch9/1
  Constant11/1 -> Switch9/2
  [VinputAdd] -> Switch9/3
  Step Perturbation VRemove/1 -> Switch8/1
  Step Perturbation VAdd/1 -> Switch10/1
  Switch9/1 -> Variable DC Source/1(Vinput)
  [VinputRemove] -> Variable DC Source/3(VinputRemove)
  [VinputAdd] -> Variable DC Source/2(VinputAdd)
  connections:
  V+/RConn1 -- Variable DC Source/RConn1
  V-/RConn1 -- Variable DC Source/RConn2

== system bObserver/ROSMO_ROSLSO/Boost Converter Circuit/Output Resistance ==
  Constant1 : Constant  Value=LoadAddSwitch
  Constant5 : Constant  Value=LoadRemoveSwitch
  Logical Operator3 : Logic  Operator=NOT  AllPortsSameDT=off  OutDataTypeStr=boolean
  Sem Disturbio : Constant
  "Sem Disturbio  " : Constant  Value=0
  Step Perturbation : PhdLibrary/Step Perturbation  SignalSwitch=LoadAddSignalSwitch  InitialMagnitude=0  InitialTime=LoadAddTime  Magnitude=1  Duration=0.1
      settings: SourceProductName=Phd Diego
  Step Perturbation1 : PhdLibrary/Step Perturbation  SignalSwitch=LoadRemoveSignalSwitch  InitialMagnitude=0  InitialTime=LoadRemoveTime  Magnitude=1  Duration=0.1
      settings: SourceProductName=Phd Diego
  Subsystem : Subsystem  mask(Variant Resistance){Ro=0, LoadAddResistor=0, LoadRemoveResistor=0}
      mask prompts: Ro "Output resistance:"; LoadAddResistor "Addtional resistance:"; LoadRemoveResistor "Resistance reduction:"
      mask help: Variant resistor according to the input signal
  Switch1 : Switch  Criteria=u2 ~= 0
  Switch5 : Switch  Criteria=u2 ~= 0
  Ro+ : PMIOPort  Side=Right
  Ro- : PMIOPort  Port=2  Side=Right
  wires:
  Constant5/1 -> Switch5/2
  Constant1/1 -> Switch1/2
  "Sem Disturbio  "/1 -> Switch5/3
  Switch1/1 -> Subsystem/1(RserieInput)
  Sem Disturbio/1 -> Switch1/3
  Step Perturbation/1 -> Logical Operator3/1
  Logical Operator3/1 -> Switch1/1
  Step Perturbation1/1 -> Switch5/1
  Switch5/1 -> Subsystem/2(Rparallelinput)
  connections:
  Ro+/RConn1 -- Subsystem/RConn1
  Ro-/RConn1 -- Subsystem/RConn2

== system bObserver/ROSMO_ROSLSO/Fault Identification/Anti false alarm ==
  alarm : Inport
  x_hat_iL : Inport  Port=2
  xe : Inport  Port=3
  e_s_signal : Inport  Port=4
  AND : Logic  IconShape=distinctive  AllPortsSameDT=off  OutDataTypeStr=boolean
  AND1 : Logic  IconShape=distinctive  AllPortsSameDT=off  OutDataTypeStr=boolean
  Constant : Constant  Value=50
  Constant7 : Constant  Value=2
  Constant8 : Constant
  Delay : Delay  DelayLength=1
  Demux10 : Demux  Outputs=2
  Demux3 : Demux  Outputs=2
  Equal : RelationalOperator  Operator===  OutDataTypeStr=boolean  RndMeth=Simplest
  GreaterThan : RelationalOperator  Operator=>  OutDataTypeStr=boolean  RndMeth=Simplest
  IC4 : InitialCondition
  Sum : Sum  Inputs=|++
  Switch : Switch
  Terminator : Terminator
  Terminator1 : Terminator
  enable : Outport
  wires:
  IC4/1 -> Switch/3
  [e_s_signal] -> IC4/1
  AND/1 -> Delay/1
  Constant/1 -> Sum/1
  AND1/1 -> AND/1
  Sum/1 -> GreaterThan/2
  GreaterThan/1 -> AND/2
  Delay/1 -> Switch/2
  Demux3/1 -> GreaterThan/1
  Constant8/1 -> Equal/1
  Equal/1 -> AND1/2
  Demux10/1 -> Sum/2
  Constant7/1 -> Switch/1
  Demux10/2 -> Terminator1/1
  x_hat_iL/1 -> Demux3/1
  Demux3/2 -> Terminator/1
  xe/1 -> Demux10/1
  alarm/1 -> AND1/1
  e_s_signal/1 -> [e_s_signal], Equal/2
  Switch/1 -> enable/1

== system bObserver/ROSMO_ROSLSO/Fault Identification/AntiFalseAlarm ==
  PRNN : Inport
  Alarm : Inport  Port=2
  Constant7 : Constant
  FaultDetecition1 : Switch  Criteria=u2 > Threshold
  Product1 : Product
  Step1 : Step  Time=AlarmDeadTime  SampleTime=0
  FaultClass : Outport
  AlarmOut : Outport  Port=2
  wires:
  PRNN/1 -> FaultDetecition1/1
  Constant7/1 -> FaultDetecition1/3
  Step1/1 -> Product1/1
  Alarm/1 -> Product1/2
  FaultDetecition1/1 -> FaultClass/1
  Product1/1 -> AlarmOut/1, FaultDetecition1/2

== system bObserver/ROSMO_ROSLSO/Fault Identification/Pattern Recognition Neural Network1 ==
  Input : Inport  PortDimensions=3
      mask Display: e = 0.06;c1 = [120 230 180]/255;c2 = ([120 230 180]+0)/(256+128);c3 = ([120 230 180]+128)/(256+128);patch([0 1 1 0],[0 0 1 1],c1);patch([0 1 1 1-e 1-e 0+e],[0 0 1 1-e 0+e 0+e],c2);patch([0 0 1 1-e 0+e 0+e],[0 1 1 1-e 1-e 0+e],c3);plot([0 1 1 0 0],[0 0 1 1 0]);
  Layer 1 : Subsystem
      mask Display: e = 0.06;c1 = [120 150 230]/255;c2 = ([120 150 230]+0)/383;c3 = ([120 150 230]+128)/383;patch([0 1 1 0],[0 0 1 1],c1);patch([0 1 1 1-e 1-e 0+e],[0 0 1 1-e 0+e 0+e],c2);patch([0 0 1 1-e 0+e 0+e],[0 1 1 1-e 1-e 0+e],c3);plot([0 1 1 0 0],[0 0 1 1 0]);
  Layer 2 : Subsystem
      mask Display: e = 0.06;c1 = [120 150 230]/255;c2 = ([120 150 230]+0)/383;c3 = ([120 150 230]+128)/383;patch([0 1 1 0],[0 0 1 1],c1);patch([0 1 1 1-e 1-e 0+e],[0 0 1 1-e 0+e 0+e],c2);patch([0 0 1 1-e 0+e 0+e],[0 1 1 1-e 1-e 0+e],c3);plot([0 1 1 0 0],[0 0 1 1 0]);
  Process Input 1 : Subsystem
      mask Display: e = 0.06;c1 = [120 150 230]/255;c2 = ([120 150 230]+0)/383;c3 = ([120 150 230]+128)/383;patch([0 1 1 0],[0 0 1 1],c1);patch([0 1 1 1-e 1-e 0+e],[0 0 1 1-e 0+e 0+e],c2);patch([0 0 1 1-e 0+e 0+e],[0 1 1 1-e 1-e 0+e],c3);plot([0 1 1 0 0],[0 0 1 1 0]);
  Process Output 1 : Subsystem
      mask Display: e = 0.06;c1 = [120 150 230]/255;c2 = ([120 150 230]+0)/383;c3 = ([120 150 230]+128)/383;patch([0 1 1 0],[0 0 1 1],c1);patch([0 1 1 1-e 1-e 0+e],[0 0 1 1-e 0+e 0+e],c2);patch([0 0 1 1-e 0+e 0+e],[0 1 1 1-e 1-e 0+e],c3);plot([0 1 1 0 0],[0 0 1 1 0]);
  Output : Outport  InitialOutput=[0;0;0;0;0]
      mask Display: e = 0.06;c1 = [120 230 180]/255;c2 = ([120 230 180]+0)/(256+128);c3 = ([120 230 180]+128)/(256+128);patch([0 1 1 0],[0 0 1 1],c1);patch([0 1 1 1-e 1-e 0+e],[0 0 1 1-e 0+e 0+e],c2);patch([0 0 1 1-e 0+e 0+e],[0 1 1 1-e 1-e 0+e],c3);plot([0 1 1 0 0],[0 0 1 1 0]);
  wires:
  Input/1 -> Process Input 1/1(x)
  Process Output 1/1(y) -> Output/1
  Process Input 1/1(p) -> Layer 1/1("p{1}")
  Layer 1/1("a{1}") -> [feedback1]
  [feedback1] -> Layer 2/1("a{1} ")
  Layer 2/1("a{2}") -> Process Output 1/1(a)

== system bObserver/ROSMO_ROSLSO/SMO/ErrorGenerator ==
  y_e_tilde : Inport
  y_e_tilde_hat : Inport  Port=2
  AND : Logic  IconShape=distinctive  AllPortsSameDT=off  OutDataTypeStr=boolean
  Compare To Zero : simulink/Logic and Bit Operations/Compare To Zero  relop=~=  OutDataTypeStr=boolean
  Constant1 : Constant  Value=[0;0]
  Demux : Demux  Outputs=2
  If : If  IfExpression=u1 ~= 0
  If Action Subsystem : Subsystem  TreatAsAtomicUnit=on
  If Action Subsystem1 : Subsystem  TreatAsAtomicUnit=on
  Merge : Merge  InitialOutput=[0;0]
  Sum : Sum  Inputs=|+-
  e_y : Outport
  v : Outport  Port=2
  wires:
  y_e_tilde/1 -> Sum/1
  y_e_tilde_hat/1 -> Sum/2
  Sum/1 -> Compare To Zero/1, e_y/1, [e_y]
  If/1 -> If Action Subsystem/Action
  If/2 -> If Action Subsystem1/Action
  [e_y] -> If Action Subsystem/1(e_y)
  Constant1/1 -> If Action Subsystem1/1(e_y)
  If Action Subsystem/1(v) -> Merge/1
  If Action Subsystem1/1(v) -> Merge/2
  Demux/1 -> AND/1
  Demux/2 -> AND/2
  AND/1 -> If/1
  Merge/1 -> v/1
  Compare To Zero/1 -> Demux/1

== system bObserver/ROSMO_ROSLSO/SMO/Sliding Mode Observer 5 ==
  ey : Inport
  v : Inport  Port=2
  sigma : Inport  Port=3
  C : Constant  Value=Ctilde1
  ObserverDynamics : Subsystem
  Product : Product  Multiplication=Matrix(*)
  ey_out : Outport
  y_e_tilde_hat : Outport  Port=2
  wires:
  Product/1 -> y_e_tilde_hat/1
  C/1 -> Product/1
  ObserverDynamics/1(e_tilde_hat) -> Product/2
  sigma/1 -> ObserverDynamics/3(sigma)
  ey/1 -> ey_out/1, ObserverDynamics/1(ey)
  v/1 -> ObserverDynamics/2(v)

== system bObserver/Slding Mode/Augmented Error Generator/z1 ==
  z_dot : Inport
  Constant1 : Constant  Value=[0;0]  VectorParams1D=off
  Gain2 : Gain  Gain=Cmatrix  Multiplication=Matrix(K*u) (u vector)
  Integrator6 : Integrator  InitialConditionSource=external
  z : Outport
  wires:
  Gain2/1 -> Integrator6/1
  Integrator6/1 -> z/1
  z_dot/1 -> Gain2/1
  Constant1/1 -> Integrator6/2

== system bObserver/Slding Mode/Boost Converter/ConversorBoost ==
  sigma : Inport
  C : powerlib/Elements/Series RLC Branch  LConnTagsString=__new0  RConnTagsString=__new0  BranchType=C  Resistance=1  Inductance=1e-3  SetiL0=off  InitialCurrent=0  Capacitance=C  Setx0=on  InitialVoltage=0  Measurements=None
  Ground : powerlib/Elements/Ground  LConnTagsString=a
  L : powerlib/Elements/Series RLC Branch  LConnTagsString=__new0  RConnTagsString=__new0  BranchType=L  Resistance=1  Inductance=L  SetiL0=on  InitialCurrent=0  Capacitance=1e-6  Setx0=off  InitialVoltage=0  Measurements=None
  R : powerlib/Elements/Series RLC Branch  LConnTagsString=__new0  RConnTagsString=__new0  BranchType=R  Resistance=R  Inductance=1e-3  SetiL0=off  InitialCurrent=0  Capacitance=1e-6  Setx0=off  InitialVoltage=0  Measurements=None
  Ro : powerlib/Elements/Series RLC Branch  LConnTagsString=__new0  RConnTagsString=__new0  BranchType=R  Resistance=Ro  Inductance=1e-3  SetiL0=off  InitialCurrent=0  Capacitance=1e-6  Setx0=off  InitialVoltage=0  Measurements=None
  S1 : powerlib/Power Electronics/Mosfet  Ron=0.0000001  Lon=0  Rd=0.000000001  Vfd=0  IC=0  Rs=1e5  Cs=inf  Measurements=on
  S2 : powerlib/Power Electronics/Diode  Ron=0.000001  Lon=0  Vf=0  IC=0  UseSnubber=off  Rs=0  Cs=0  Measurements=on
  Tensão Ve1 : Display
  Terminator : Terminator
  Terminator4 : Terminator
  Voltage Measurement : powerlib/Measurements/Voltage Measurement  PhasorSimulation=off  OutputType=Complex  PSBequivalent=0
  Voltage Measurement1 : powerlib/Measurements/Voltage Measurement  PhasorSimulation=off  OutputType=Complex  PSBequivalent=0
  u : powerlib/Electrical Sources/DC Voltage Source  Amplitude=u  Measurements=None
  Vcoutput : Outport
  Vu : Outport  Port=2
  wires:
  sigma/1 -> S1/1
  Voltage Measurement/1 -> Vcoutput/1
  Voltage Measurement1/1 -> Vu/1, Tensão Ve1/1
  S1/1 -> Terminator/1
  S2/1 -> Terminator4/1
  connections:
  S1/LConn1 -- L/RConn1 -- S2/LConn1
  C/RConn1 -- Ro/RConn1 -- Ground/LConn1 -- u/LConn1 -- Voltage Measurement1/LConn2 -- S1/RConn1 -- Voltage Measurement/LConn2
  Voltage Measurement1/LConn1 -- u/RConn1 -- R/LConn1
  L/LConn1 -- R/RConn1
  Ro/LConn1 -- Voltage Measurement/LConn1 -- C/LConn1 -- S2/RConn1

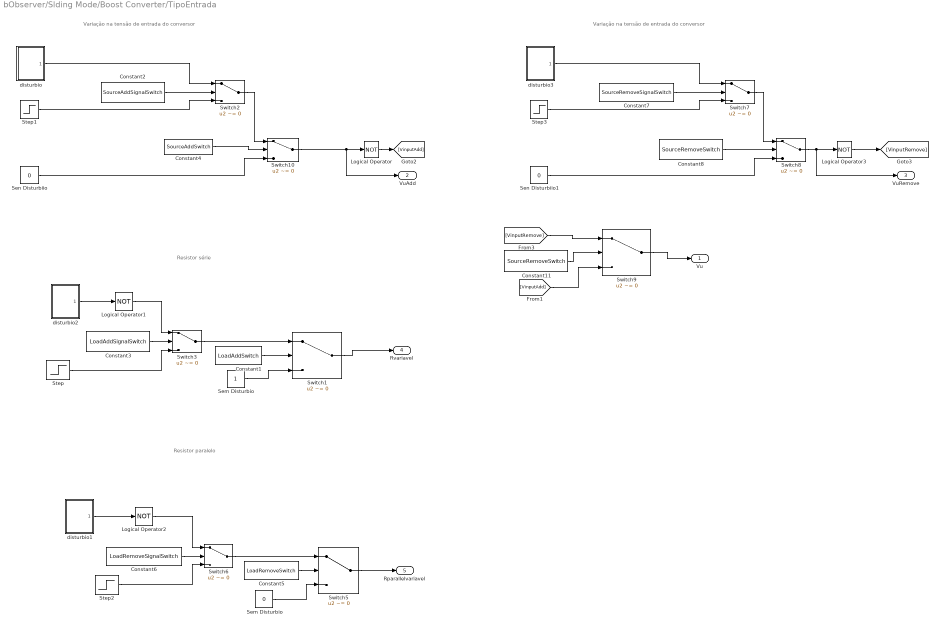
== system bObserver/Slding Mode/Boost Converter/TipoEntrada ==
  note: Variação na tensão de entrada do conversor
  note: Resistor série
  note: Resistor paralelo
  note: Variação na tensão de entrada do conversor
  Constant1 : Constant  Value=LoadAddSwitch
  Constant11 : Constant  Value=SourceRemoveSwitch
  Constant2 : Constant  Value=SourceAddSignalSwitch
  Constant3 : Constant  Value=LoadAddSignalSwitch
  Constant4 : Constant  Value=SourceAddSwitch
  Constant5 : Constant  Value=LoadRemoveSwitch
  Constant6 : Constant  Value=LoadRemoveSignalSwitch
  Constant7 : Constant  Value=SourceRemoveSignalSwitch
  Constant8 : Constant  Value=SourceRemoveSwitch
  Logical Operator{,1..3} (4 alike) : Logic  Operator=NOT  AllPortsSameDT=off  OutDataTypeStr=boolean
  Sem Disturbio : Constant
  "Sem Disturbio  " : Constant  Value=0
  Sen Disturbiio : Constant  Value=0
  Sen Disturbiio1 : Constant  Value=0
  Step : Step  Time=LoadAddTime  Before=1  After=0  SampleTime=0
  Step1 : Step  Time=SourceAddTime  SampleTime=0
  Step2 : Step  Time=LoadRemoveTime  SampleTime=0
  Step3 : Step  Time=SourceRemoveTime  SampleTime=0
  Switch{1..3,5..10} (9 alike) : Switch  Criteria=u2 ~= 0
  disturbio : Subsystem
  disturbio1 : Subsystem
  disturbio2 : Subsystem
  disturbio3 : Subsystem
  Vu : Outport
  VuAdd : Outport  Port=2
  VuRemove : Outport  Port=3
  "Rvariavel " : Outport  Port=4
  "Rparallelvariavel " : Outport  Port=5
  wires:
  Sen Disturbiio/1 -> Switch10/3
  Constant4/1 -> Switch10/2
  Constant1/1 -> Switch1/2
  Switch1/1 -> "Rvariavel "/1
  Constant2/1 -> Switch2/2
  Constant3/1 -> Switch3/2
  Switch2/1 -> Switch10/1
  disturbio2/1(disturbio) -> Logical Operator1/1
  Switch3/1 -> Switch1/1
  Sem Disturbio/1 -> Switch1/3
  Switch6/1 -> Switch5/1
  disturbio1/1(disturbio) -> Logical Operator2/1
  Constant6/1 -> Switch6/2
  "Sem Disturbio  "/1 -> Switch5/3
  Switch5/1 -> "Rparallelvariavel "/1
  Constant5/1 -> Switch5/2
  disturbio/1(disturbio) -> Switch2/1
  Step1/1 -> Switch2/3
  Logical Operator1/1 -> Switch3/1
  Step/1 -> Switch3/3
  Step2/1 -> Switch6/3
  Logical Operator2/1 -> Switch6/1
  disturbio3/1(disturbio) -> Switch7/1
  Constant8/1 -> Switch8/2
  Constant7/1 -> Switch7/2
  Switch8/1 -> VuRemove/1, Logical Operator3/1
  Sen Disturbiio1/1 -> Switch8/3
  Switch7/1 -> Switch8/1
  Step3/1 -> Switch7/3
  [VinputAdd] -> Switch9/3
  Constant11/1 -> Switch9/2
  Switch10/1 -> VuAdd/1, Logical Operator/1
  Switch9/1 -> Vu/1
  Logical Operator/1 -> [VinputAdd]
  Logical Operator3/1 -> [VinputRemove]
  [VinputRemove] -> Switch9/1

== system bObserver/Slding Mode/Controlador1/SlidingSurface ==
  S : Inport
  ep : Inport  Port=2
  Abs : Abs
  GreaterThan : RelationalOperator  Operator=>  OutDataTypeStr=boolean  RndMeth=Simplest
  If : If  IfExpression=u1 ~= 0
  If Action Subsystem : Subsystem  TreatAsAtomicUnit=on
  If Action Subsystem2 : Subsystem  TreatAsAtomicUnit=on
  Merge1 : Merge
  d : Outport
  wires:
  If Action Subsystem2/1(d) -> Merge1/2
  [S] -> If Action Subsystem/1(S), If Action Subsystem2/1(S)
  If/2 -> If Action Subsystem2/Action
  If/1 -> If Action Subsystem/Action
  [ep] -> If Action Subsystem2/2(ep)
  S/1 -> [S], Abs/1
  If Action Subsystem/1(d) -> Merge1/1
  Abs/1 -> GreaterThan/1
  GreaterThan/1 -> If/1
  Merge1/1 -> d/1
  ep/1 -> [ep], GreaterThan/2

== system bObserver/Slding Mode/D(f_s)/Subsystem ==
  input : Inport
  FaultStep : Inport  Port=2
  NoiseStep : Inport  Port=3
  FaultSwtich : Inport  Port=4
  NoiseFaultSwitch : Inport  Port=5
  FaultFactor : Inport  Port=6
  Constant11 : Constant  Value=0
  Constant9 : Constant  Value=0
  Product : Product
  Subsystem : Subsystem
  Switch{9..11,13} (4 alike) : Switch  Criteria=u2 ~= 0
  iLFault Switch : MultiPortSwitch  DataPortOrder=Zero-based contiguous  DataPortForDefault=Additional data port  zeroidx=on
  output : Outport
  wires:
  input/1 -> Product/1, Switch11/3, Switch10/3, iLFault Switch/2, iLFault Switch/5
  Constant9/1 -> Switch10/1
  Switch13/1 -> Switch9/2
  Switch9/1 -> output/1
  Switch11/1 -> iLFault Switch/4
  Constant11/1 -> Switch13/3
  iLFault Switch/1 -> Switch9/3, Subsystem/1(input)
  Switch10/1 -> iLFault Switch/3
  FaultStep/1 -> Switch10/2, Switch11/2
  NoiseStep/1 -> Switch13/1
  FaultSwtich/1 -> iLFault Switch/1
  NoiseFaultSwitch/1 -> Switch13/2
  Product/1 -> Switch11/1
  FaultFactor/1 -> Product/2
  Subsystem/1(noiseOutput) -> Switch9/1

== system bObserver/Slding Mode/D(f_s)/Subsystem2 ==
  input : Inport
  FaultStep : Inport  Port=2
  NoiseStep : Inport  Port=3
  FaultSwtich : Inport  Port=4
  NoiseFaultSwitch : Inport  Port=5
  FaultFactor : Inport  Port=6
  Constant11 : Constant  Value=0
  Constant9 : Constant  Value=0
  Product : Product
  Subsystem : Subsystem
  Switch10 : Switch  Criteria=u2 ~= 0
  Switch11 : Switch  Criteria=u2 ~= 0
  Switch13 : Switch  Criteria=u2 ~= 0
  Switch9 : Switch  Criteria=u2 ~= 0  ZeroCross=off
  iLFault Switch : MultiPortSwitch  DataPortOrder=Zero-based contiguous  DataPortForDefault=Additional data port  zeroidx=on
  output : Outport
  wires:
  input/1 -> Product/1, Switch11/3, iLFault Switch/2, Switch10/3, iLFault Switch/5
  Constant9/1 -> Switch10/1
  Switch13/1 -> Switch9/2
  Switch9/1 -> output/1
  Switch11/1 -> iLFault Switch/4
  Constant11/1 -> Switch13/3
  iLFault Switch/1 -> Switch9/3, Subsystem/1(input)
  Switch10/1 -> iLFault Switch/3
  FaultStep/1 -> Switch11/2, Switch10/2
  NoiseStep/1 -> Switch13/1
  FaultSwtich/1 -> iLFault Switch/1
  NoiseFaultSwitch/1 -> Switch13/2
  FaultFactor/1 -> Product/2
  Product/1 -> Switch11/1
  Subsystem/1(noiseOutput) -> Switch9/1
